simulink model "Remus_pitch_control_240821"  (R2023b)
settings: Solver=ode1  StartTime=0.0  StopTime=T_final  FixedStep=Ts  RelTol=1e-3
values from neighbouring files (symbols this model uses):
  A = [-1.36757087013 -0.0298365607614 1.00305051334e-21 -2.85933126392 0.119442498277 -1.97014537421e-22 1 0 0 0 0 0 ... (144 elements, 12x12)]    [linmodel_u_2kts.mat]
  B = [0 -0.0899434384233 0 -0.353204156384 0 0.57859211058 0 0 0 0 0 0 ... (36 elements, 12x3)]    [linmodel_u_2kts.mat]
  C = [1 0 0 0 0 0 0 0 0 0 0 0 ... (144 elements, 12x12)]    [linmodel_u_2kts.mat]
  D = [0 0 0 0 0 0 0 0 0 0 0 0 ... (36 elements, 12x3)]    [linmodel_u_2kts.mat]
  Kd_theta = 0.115    [compare_PID.m]
  Ki_theta = 0.38    [compare_PID.m]
  Kp_theta = 0.6    [compare_PID.m]
  stern_max = 45    [compare_PID.m]
  Ts = 0.01    [compare_PID.m]
  x0 = [2 -4.48954579629e-15 -5.26283161463e-21 1.99783697576e-20 -6.52845367291e-21 7.55477241533e-22 2.13618802829e-15 -1.75591256947e-16 1.82878054643e-16 0.109446709475 0 0]    [trim_u_2kts.mat]
undefined symbols (not defined in the file or in its folder): Ki_theta2, Kn, Kp_theta2
libraries: simulink_extras x12, simulink x1, slpidlib x1
settings Model: Creator=ADMIN  LastModifiedBy=ADMIN
settings DebuggingCC: UnconnectedInputMsg=warning  UnconnectedOutputMsg=warning  UnconnectedLineMsg=warning
settings ModelReferenceCC: EnableRefExpFcnMdlSchedulingChecks=on
settings RTWCC: DLArmComputeVersion=19.05

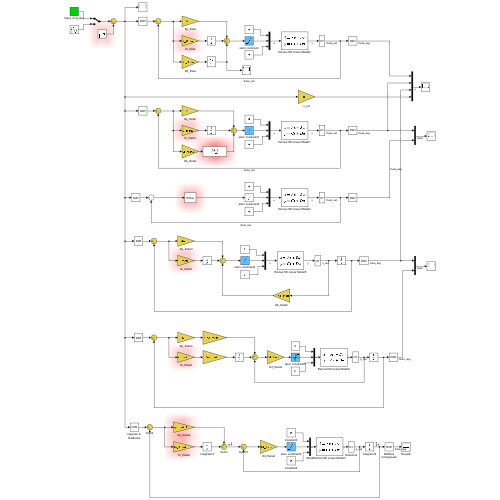
[thumbnail: Simulink's stored preview of the top-level diagram]
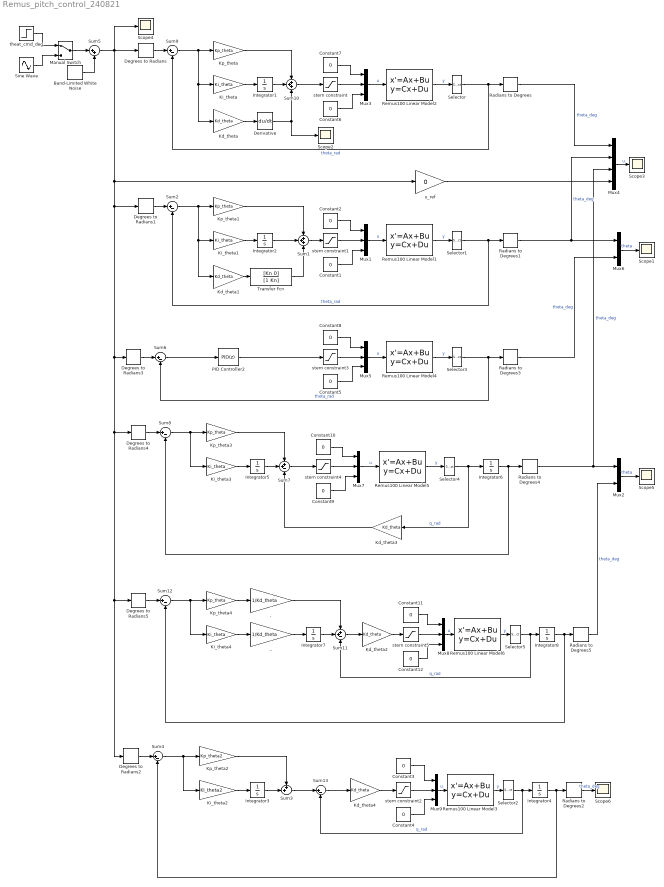
== system Remus_pitch_control_240821 ==
  . : Gain  Gain=1/Kd_theta  SaturateOnIntegerOverflow=on  OutDataTypeStr=Inherit: Same as input  ParamDataTypeStr=Inherit: Same as input
  .. : Gain  Gain=1/Kd_theta  SaturateOnIntegerOverflow=on  OutDataTypeStr=Inherit: Same as input  ParamDataTypeStr=Inherit: Same as input
  Band-Limited White Noise : simulink/Sources/Band-Limited White Noise  Cov=[0.00001]  Ts=Ts  seed=[23341]
  Constant{1..12} (12 alike) : Constant  Value=0  OutDataTypeStr=double
  Degrees to Radians{,1..5} (6 alike) : simulink_extras/Transformations/Degrees to Radians
  Derivative : Derivative
  Integrator{1..8} (8 alike) : Integrator
  Kd_theta{,1..4} (5 alike) : Gain  Gain=Kd_theta  SaturateOnIntegerOverflow=on  OutDataTypeStr=Inherit: Same as input  ParamDataTypeStr=Inherit: Same as input
  Ki_theta{,1,3..4} (4 alike) : Gain  Gain=Ki_theta  SaturateOnIntegerOverflow=on  OutDataTypeStr=Inherit: Same as input  ParamDataTypeStr=Inherit: Same as input
  Ki_theta2 : Gain  Gain=Ki_theta2  SaturateOnIntegerOverflow=on  OutDataTypeStr=Inherit: Same as input  ParamDataTypeStr=Inherit: Same as input
  Kp_theta{,1,3..4} (4 alike) : Gain  Gain=Kp_theta  SaturateOnIntegerOverflow=on  OutDataTypeStr=Inherit: Same as input  ParamDataTypeStr=Inherit: Same as input
  Kp_theta2 : Gain  Gain=Kp_theta2  SaturateOnIntegerOverflow=on  OutDataTypeStr=Inherit: Same as input  ParamDataTypeStr=Inherit: Same as input
  Manual Switch : ManualSwitch
  Mux{1,3,5,7..9} (6 alike) : Mux  Inputs=3
  Mux2 : Mux  Inputs=2
  Mux4 : Mux
  Mux6 : Mux  Inputs=2
  PID Controller2 : slpidlib/PID Controller  Controller=PID  Form=Parallel  TimeDomain=Discrete-time  UseExternalTs=off  SampleTime=Ts  IntegratorMethod=Forward Euler  FilterMethod=Forward Euler  ControllerParametersSource=internal  P=Kp_theta  I=Ki_theta  UseKiTs=off  D=Kd_theta  N=Kn  UseFilter=on  TunerSelectOption=Transfer Function Based (PID Tuner App)  InitialConditionSource=internal  InitialConditionForIntegrator=0  InitialConditionForFilter=0  DifferentiatorICPrevScaledInput=0  ExternalReset=none  TrackingMode=off  Kt=1  LimitOutput=off  SatLimitsSource=internal  UpperSaturationLimit=inf  LowerSaturationLimit=-inf  LinearizeAsGain=on  AntiWindupMode=none  Kb=1  LimitIntegrator=off  UpperIntegratorSaturationLimit=inf  LowerIntegratorSaturationLimit=-inf  POutMin=[]  POutMax=[]  IOutMin=[]  IOutMax=[]  DOutMin=[]  DOutMax=[]  NOutMin=[]  NOutMax=[]  SumOutMin=[]  SumOutMax=[]  SaturationOutMin=[]  SaturationOutMax=[]  PParamMin=[]  PParamMax=[]  IParamMin=[]  IParamMax=[]  DParamMin=[]  DParamMax=[]  NParamMin=[]  NParamMax=[]  KbParamMin=[]  KbParamMax=[]  KtParamMin=[]  KtParamMax=[]  KbOutMin=[]  KbOutMax=[]  KtOutMin=[]  KtOutMax=[]  IntegratorOutMin=[]  IntegratorOutMax=[]  FilterOutMin=[]  FilterOutMax=[]  SumI1OutMin=[]  SumI1OutMax=[]  SumI2OutMin=[]  SumI2OutMax=[]  SumI3OutMin=[]  SumI3OutMax=[]  SumI4OutMin=[]  SumI4OutMax=[]  SumDOutMin=[]  SumDOutMax=[]  DifferentiatorOutMin=[]  DifferentiatorOutMax=[]  FilterDiffOutCoefMin=[]  FilterDiffOutCoefMax=[]  ReciprocalOutMin=[]  ReciprocalOutMax=[]  SumDenOutMin=[]  SumDenOutMax=[]  SumNumOutMin=[]  SumNumOutMax=[]  DivideOutMin=[]  DivideOutMax=[]  UdiffTsProdOutMin=[]  UdiffTsProdOutMax=[]  NTsProdOutMin=[]  NTsProdOutMax=[]  UintegralTsProdOutMin=[]  UintegralTsProdOutMax=[]  UngainTsProdOutMin=[]  UngainTsProdOutMax=[]  ClampingZeroOutDataTypeStr=Inherit: Inherit via back propagation  ClampingZeroOutMin=[]  ClampingZeroOutMax=[]  FilterDenConstantOutDataTypeStr=Inherit: Inherit via back propagation  FilterDenConstantOutMin=[]  FilterDenConstantOutMax=[]  PCopyOutDataTypeStr=Inherit: Inherit via back propagation  PCopyOutMin=[]  PCopyOutMax=[]  NCopyOutDataTypeStr=Inherit: Inherit via back propagation  NCopyOutMin=[]  NCopyOutMax=[]  IntegratorContinuousStateAttributes=''  IntegratorStateMustResolveToSignalObject=off  IntegratorRTWStateStorageClass=Auto  FilterContinuousStateAttributes=''  FilterStateMustResolveToSignalObject=off  FilterRTWStateStorageClass=Auto  ParallelPVariant=InternalParameters  IdealPVariant=Disabled  IVariant=InternalParameters  DVariant=InternalParameters  IntegratorVariant=Discrete  SatVariant=Disabled  AWVariant=Passthrough  PCopyVariant=Disabled  TRVariant=Disabled  FdbkBlocksVariant=Forward  IdealPFdbkVariant=Disabled  SatFdbkVariant=Disabled  DerivativeFilterVariant=ForwardEulerFilter  NVariant=InternalParameters  NCopyVariant=Disabled  FilterICVariant=InternalICsFilter  IntegratorICVariant=InternalICs  ExternalResetVariant=Disabled  TRSumVariant=Passthrough  SumFdbkVariant=Disabled  SumVariant=Sum_PID  TsampFilterVariant=InternalTs  TsampNgainVariant=Passthrough  TsampIntegralVariant=Disabled_SignalSpec  ExternalSaturationOutDataTypeStr=Inherit: Same as second input
  Radians to Degrees{,1..5} (6 alike) : simulink_extras/Transformations/Radians to Degrees
  Remus100 Linear Model{1..6} (6 alike) : StateSpace  A=A  B=B  C=C  D=D  InitialCondition=x0*0
  Scope{1..6} (6 alike) : Scope
  Selector : Selector  InputPortWidth=12  IndexOptions=Index vector (dialog)  Indices=11  OutputSizes=1
  Selector1 : Selector  InputPortWidth=12  IndexOptions=Index vector (dialog)  Indices=11  OutputSizes=1
  Selector2 : Selector  InputPortWidth=12  IndexOptions=Index vector (dialog)  Indices=5  OutputSizes=1
  Selector3 : Selector  InputPortWidth=12  IndexOptions=Index vector (dialog)  Indices=11  OutputSizes=1
  Selector4 : Selector  InputPortWidth=12  IndexOptions=Index vector (dialog)  Indices=5  OutputSizes=1
  Selector5 : Selector  InputPortWidth=12  IndexOptions=Index vector (dialog)  Indices=5  OutputSizes=1
  Sine Wave : Sin  SampleTime=0
  Sum1 : Sum  Inputs=+++  InputSameDT=on  SaturateOnIntegerOverflow=on  OutDataTypeStr=Inherit: Same as first input
  Sum10 : Sum  Inputs=+++  InputSameDT=on  SaturateOnIntegerOverflow=on  OutDataTypeStr=Inherit: Same as first input
  Sum11 : Sum  Inputs=++-  InputSameDT=on  SaturateOnIntegerOverflow=on  OutDataTypeStr=Inherit: Same as first input
  Sum{2,4,6,8..9,12..13} (7 alike) : Sum  Inputs=|+-  InputSameDT=on  SaturateOnIntegerOverflow=on  OutDataTypeStr=Inherit: Same as first input
  Sum3 : Sum  Inputs=++|  InputSameDT=on  SaturateOnIntegerOverflow=on  OutDataTypeStr=Inherit: Same as first input
  Sum5 : Sum  Inputs=|++  InputSameDT=on  SaturateOnIntegerOverflow=on  OutDataTypeStr=Inherit: Same as first input
  Sum7 : Sum  Inputs=++-  InputSameDT=on  SaturateOnIntegerOverflow=on  OutDataTypeStr=Inherit: Same as first input
  Transfer Fcn : TransferFcn  Numerator=[Kn 0]  Denominator=[1 Kn]
  stern constraint{,1..5} (6 alike) : Saturate  UpperLimit=stern_max*deg2rad  LowerLimit=-stern_max*deg2rad
  theat_cmd_deg : Step  Time=0  SampleTime=0
  u_ref : Gain  Gain=0  SaturateOnIntegerOverflow=on  OutDataTypeStr=Inherit: Same as input  ParamDataTypeStr=Inherit: Same as input
  wires:
  Mux3/1 -> Remus100 Linear Model2/1  "u"
  Constant6/1 -> Mux3/3
  stern constraint/1 -> Mux3/2
  Constant7/1 -> Mux3/1
  Sum9/1 -> Kp_theta/1, Kd_theta/1, Ki_theta/1
  Degrees to Radians/1 -> Sum9/1
  Sum10/1 -> stern constraint/1
  Radians to Degrees/1 -> Mux4/1  "theta_deg"
  Selector/1 -> Radians to Degrees/1, Sum9/2  "theta_rad"
  Remus100 Linear Model2/1 -> Selector/1  "y"
  Integrator1/1 -> Sum10/2
  Kp_theta/1 -> Sum10/1
  Ki_theta/1 -> Integrator1/1
  Kd_theta/1 -> Derivative/1
  Derivative/1 -> Sum10/3, Scope2/1
  stern constraint1/1 -> Mux1/2
  Kp_theta1/1 -> Sum1/1
  Kd_theta1/1 -> Transfer Fcn/1
  Ki_theta1/1 -> Integrator2/1
  Transfer Fcn/1 -> Sum1/3
  theat_cmd_deg/1 -> Manual Switch/1
  Radians to Degrees1/1 -> Mux4/2, Mux6/1  "theta_deg"
  Sum2/1 -> Kp_theta1/1, Kd_theta1/1, Ki_theta1/1
  Constant2/1 -> Mux1/1
  Integrator2/1 -> Sum1/2
  Constant1/1 -> Mux1/3
  Degrees to Radians1/1 -> Sum2/1
  Mux1/1 -> Remus100 Linear Model1/1  "u"
  Sum1/1 -> stern constraint1/1
  Selector1/1 -> Radians to Degrees1/1, Sum2/2  "theta_rad"
  Remus100 Linear Model1/1 -> Selector1/1  "y"
  Sine Wave/1 -> Manual Switch/2
  Manual Switch/1 -> Sum5/1
  Mux4/1 -> Scope3/1  "u"
  Sum5/1 -> Scope4/1, Degrees to Radians1/1, Degrees to Radians2/1, Degrees to Radians5/1, Degrees to Radians4/1, Degrees to Radians3/1, u_ref/1, Degrees to Radians/1
  Band-Limited White Noise/1 -> Sum5/2
  Sum6/1 -> PID Controller2/1
  Mux5/1 -> Remus100 Linear Model4/1  "u"
  Constant5/1 -> Mux5/3
  stern constraint3/1 -> Mux5/2
  Selector3/1 -> Radians to Degrees3/1, Sum6/2  "theta_rad"
  Remus100 Linear Model4/1 -> Selector3/1  "y"
  Degrees to Radians3/1 -> Sum6/1
  Radians to Degrees3/1 -> Mux6/2  "theta_deg"
  Constant8/1 -> Mux5/1
  Mux6/1 -> Scope1/1  "theta"
  PID Controller2/1 -> stern constraint3/1
  u_ref/1 -> Mux4/4
  Kd_theta3/1 -> Sum7/3
  Integrator6/1 -> Sum8/2, Radians to Degrees4/1
  Sum7/1 -> stern constraint4/1
  stern constraint4/1 -> Mux7/2
  Degrees to Radians4/1 -> Sum8/1
  Kp_theta3/1 -> Sum7/1
  Ki_theta3/1 -> Integrator5/1
  Mux7/1 -> Remus100 Linear Model5/1  "u"
  Sum8/1 -> Ki_theta3/1, Kp_theta3/1
  Constant10/1 -> Mux7/1
  Integrator5/1 -> Sum7/2
  Constant9/1 -> Mux7/3
  Remus100 Linear Model5/1 -> Selector4/1  "y"
  Selector4/1 -> Integrator6/1, Kd_theta3/1  "q_rad"
  Selector5/1 -> Integrator8/1, Sum11/3  "q_rad"
  Remus100 Linear Model6/1 -> Selector5/1  "y"
  Constant12/1 -> Mux8/3
  Integrator7/1 -> Sum11/2
  Constant11/1 -> Mux8/1
  Sum12/1 -> Kp_theta4/1, Ki_theta4/1
  Mux8/1 -> Remus100 Linear Model6/1  "u"
  Ki_theta4/1 -> ../1
  Kp_theta4/1 -> ./1
  Degrees to Radians5/1 -> Sum12/1
  stern constraint5/1 -> Mux8/2
  Sum11/1 -> Kd_theta2/1
  Integrator8/1 -> Radians to Degrees5/1, Sum12/2
  Radians to Degrees4/1 -> Mux2/1, Mux4/3  "theta_deg"
  Mux2/1 -> Scope5/1  "theta"
  Radians to Degrees5/1 -> Mux2/2  "theta_deg"
  Kd_theta2/1 -> stern constraint5/1
  ./1 -> Sum11/1
  ../1 -> Integrator7/1
  Ki_theta2/1 -> Integrator3/1
  Kp_theta2/1 -> Sum3/1
  Kd_theta4/1 -> stern constraint2/1
  Integrator4/1 -> Sum4/2, Radians to Degrees2/1
  stern constraint2/1 -> Mux9/2
  Degrees to Radians2/1 -> Sum4/1
  Mux9/1 -> Remus100 Linear Model3/1  "u"
  Sum4/1 -> Ki_theta2/1, Kp_theta2/1
  Constant3/1 -> Mux9/1
  Integrator3/1 -> Sum3/2
  Constant4/1 -> Mux9/3
  Remus100 Linear Model3/1 -> Selector2/1  "y"
  Selector2/1 -> Sum13/2, Integrator4/1  "q_rad"
  Radians to Degrees2/1 -> Scope6/1  "theta_deg"
  Sum13/1 -> Kd_theta4/1
  Sum3/1 -> Sum13/1
